simulink model "mdl01"  (Simulink 7.4)
settings: Solver=ode45  StartTime=0.0  StopTime=10.0  RelTol=1e-3
libraries: NAV420Lib x4
settings Model: Creator=autopilot  LastModifiedBy=autopilot

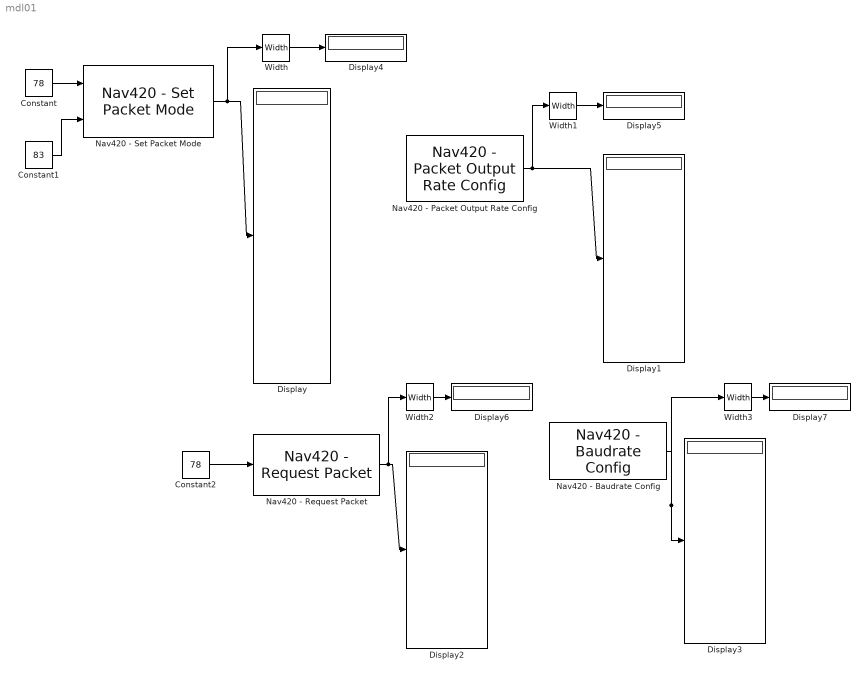
== system mdl01 ==
  Constant : Constant  Value=78  OutDataTypeMode=int8  OutDataType=fixdt(1, 16)  OutScaling=2^0  OutDataTypeStr=int8
  Constant1 : Constant  Value=83  OutDataTypeMode=int8  OutDataType=fixdt(1, 16)  OutScaling=2^0  OutDataTypeStr=int8
  Constant2 : Constant  Value=78  OutDataTypeMode=int8  OutDataType=fixdt(1, 16)  OutScaling=2^0  OutDataTypeStr=int8
  Display{,1..7} (8 alike) : Display
      Display settings: Format=hex (Stored Integer)
      Display1 settings: Format=hex (Stored Integer)
      Display2 settings: Format=hex (Stored Integer)
      Display3 settings: Format=hex (Stored Integer)
  Nav420 - Baudrate Config : NAV420Lib/Nav420 - Baudrate Config  SystemSampleTime=-1  baudrateIndex=57600  SaveConfig=off
  Nav420 - Packet Output Rate Config : NAV420Lib/Nav420 - Packet Output Rate Config  SystemSampleTime=-1  shouldSave=off  output_rate=0
  Nav420 - Request Packet : NAV420Lib/Nav420 - Request Packet  SystemSampleTime=-1
  Nav420 - Set Packet Mode : NAV420Lib/Nav420 - Set Packet Mode  SystemSampleTime=-1
  Width{,1..3} (4 alike) : Width
  wires:
  Constant/1 -> Nav420 - Set Packet Mode/1
  Constant1/1 -> Nav420 - Set Packet Mode/2
  Nav420 - Set Packet Mode/1 -> Display/1, Width/1
  Nav420 - Packet Output Rate Config/1 -> Display1/1, Width1/1
  Constant2/1 -> Nav420 - Request Packet/1
  Nav420 - Baudrate Config/1 -> Display3/1, Width3/1
  Nav420 - Request Packet/1 -> Display2/1, Width2/1
  Width2/1 -> Display6/1
  Width3/1 -> Display7/1
  Width1/1 -> Display5/1
  Width/1 -> Display4/1
